simulink subsystem "rss_pmsm_thermal_model"  (R2022b)
settings: Solver=VariableStepAuto  StartTime=0.0  StopTime=10.0  RelTol=1e-3
undefined symbols (not defined in the file): Mag_Temp, oiltemp, speed, torque, Wind_Temp
settings Model: Creator=NAH2OFO  LastModifiedBy=CAV2OFO

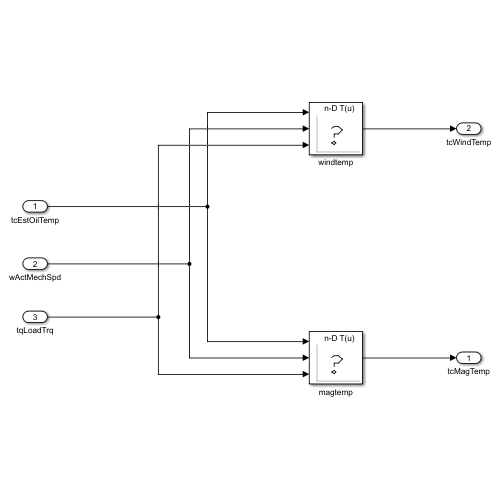
[thumbnail: Simulink's stored preview of the top-level diagram]
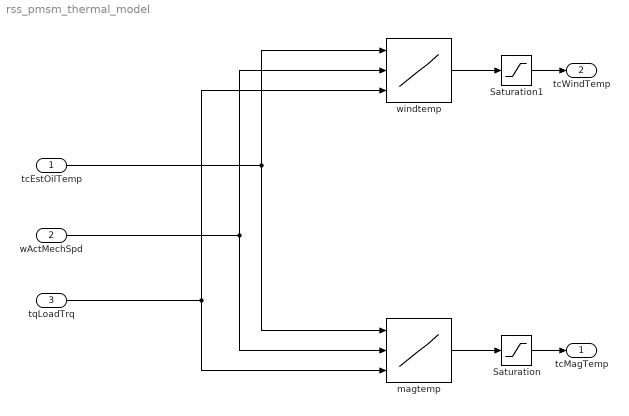
== system rss_pmsm_thermal_model ==
  tcEstOilTemp : Inport
  wActMechSpd : Inport  Port=2
  tqLoadTrq : Inport  Port=3
  Saturation : Saturate  UpperLimit=200  LowerLimit=-50
  Saturation1 : Saturate  UpperLimit=200  LowerLimit=-50
  magtemp : Lookup_n-D  NumberOfTableDimensions=3  BreakpointsForDimension1=oiltemp  BreakpointsForDimension2=speed  BreakpointsForDimension3=torque  Table=Mag_Temp  InternalRulePriority=Speed  RndMeth=Simplest
      settings: InputPortMap=u0,u1,u2
  windtemp : Lookup_n-D  NumberOfTableDimensions=3  BreakpointsForDimension1=oiltemp  BreakpointsForDimension2=speed  BreakpointsForDimension3=torque  Table=Wind_Temp  InternalRulePriority=Speed  RndMeth=Simplest
      settings: InputPortMap=u0,u1,u2
  tcMagTemp : Outport
  tcWindTemp : Outport  Port=2
  wires:
  magtemp/1 -> Saturation/1
  tqLoadTrq/1 -> windtemp/3, magtemp/3
  wActMechSpd/1 -> windtemp/2, magtemp/2
  tcEstOilTemp/1 -> windtemp/1, magtemp/1
  windtemp/1 -> Saturation1/1
  Saturation/1 -> tcMagTemp/1
  Saturation1/1 -> tcWindTemp/1
